simulink model "MLP_Final_Golden"  (R2015b)
settings: Solver=FixedStepDiscrete  SolverMode=SingleTasking  StartTime=0.0  StopTime=1e-2  RelTol=1e-3
undefined symbols (not defined in the file): input_sample_time, system_sample_time
libraries: shlslibv1 x1948
(part 1 of 11)
settings Model: synDspstartup=OK  Creator=txia13  LastModifiedBy=sshi23
settings DataIOCC: SaveOutput=off  SignalLogging=off  SaveTime=off
settings OptimizationCC: DefaultParameterBehavior=Inlined
settings DebuggingCC: AlgebraicLoopMsg=error  InheritedTsInSrcMsg=none

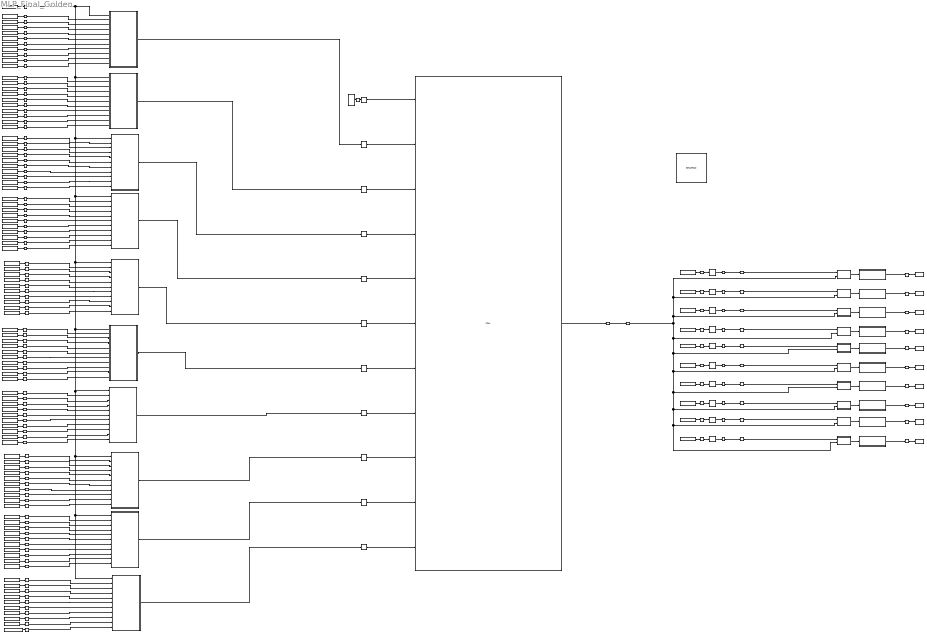
== system MLP_Final_Golden ==
  "Activation_Preparation_LoopLatency10 " : Subsystem
  Activation_Preparation_LoopLatency10 1 : Subsystem
  Activation_Preparation_LoopLatency10 2 : Subsystem
  Activation_Preparation_LoopLatency10 3 : Subsystem
  Activation_Preparation_LoopLatency10 4 : Subsystem
  Activation_Preparation_LoopLatency10 5 : Subsystem
  Activation_Preparation_LoopLatency10 6 : Subsystem
  Activation_Preparation_LoopLatency10 7 : Subsystem
  Activation_Preparation_LoopLatency10 8 : Subsystem
  Activation_Preparation_LoopLatency10 9 : Subsystem
  Counter : shlslibv1/Sources/Counter  syn_rst_port=off  syn_en_port=off  syn_ld_port=off  syn_cnt_type=Up  syn_init_val=0  syn_term_exists=on  syn_rdy_port=off  syn_term_val=9  syn_cnt_f=Automatic  syn_cnt_wl=8  syn_cnt_dt=unsigned  syn_cnt_st=BMUX_sample_time  synBlockType=primitive  synLatency=0  synBlockId=21
  Delay{1..10,21} (11 alike) : shlslibv1/Memories/Delay  syn_delay_val=7891  synBlockType=primitive  synLatency=7891  synBlockId=104
  Delay11 : shlslibv1/Memories/Delay  syn_delay_val=2  synBlockType=primitive  synLatency=2  synBlockId=104
  Delay12 : shlslibv1/Memories/Delay  syn_delay_val=12  synBlockType=primitive  synLatency=12  synBlockId=104
  Delay13 : shlslibv1/Memories/Delay  syn_delay_val=22  synBlockType=primitive  synLatency=22  synBlockId=104
  Delay14 : shlslibv1/Memories/Delay  syn_delay_val=32  synBlockType=primitive  synLatency=32  synBlockId=104
  Delay15 : shlslibv1/Memories/Delay  syn_delay_val=42  synBlockType=primitive  synLatency=42  synBlockId=104
  Delay16 : shlslibv1/Memories/Delay  syn_delay_val=52  synBlockType=primitive  synLatency=52  synBlockId=104
  Delay17 : shlslibv1/Memories/Delay  syn_delay_val=62  synBlockType=primitive  synLatency=62  synBlockId=104
  Delay18 : shlslibv1/Memories/Delay  syn_delay_val=72  synBlockType=primitive  synLatency=72  synBlockId=104
  Delay19 : shlslibv1/Memories/Delay  syn_delay_val=82  synBlockType=primitive  synLatency=82  synBlockId=104
  Delay20 : shlslibv1/Memories/Delay  syn_delay_val=92  synBlockType=primitive  synLatency=92  synBlockId=104
  From Workspace : FromWorkspace  VariableName=Input_Layer  SampleTime=input_sample_time  OutputAfterFinalValue=Setting to zero
  From Workspace1 : FromWorkspace  VariableName=Hidden_Layer_Weight1  SampleTime=input_sample_time  OutputAfterFinalValue=Setting to zero
  From Workspace10 : FromWorkspace  VariableName=Hidden_Layer_Weight5  SampleTime=input_sample_time  OutputAfterFinalValue=Setting to zero
  From Workspace102 : FromWorkspace  VariableName=Hidden_Layer_Weight51  SampleTime=input_sample_time  OutputAfterFinalValue=Setting to zero
  From Workspace103 : FromWorkspace  VariableName=Hidden_Layer_Weight55  SampleTime=input_sample_time  OutputAfterFinalValue=Setting to zero
  From Workspace106 : FromWorkspace  VariableName=Hidden_Layer_Weight56  SampleTime=input_sample_time  OutputAfterFinalValue=Setting to zero
  From Workspace107 : FromWorkspace  VariableName=Hidden_Layer_Weight58  SampleTime=input_sample_time  OutputAfterFinalValue=Setting to zero
  From Workspace109 : FromWorkspace  VariableName=Hidden_Layer_Weight59  SampleTime=input_sample_time  OutputAfterFinalValue=Setting to zero
  From Workspace111 : FromWorkspace  VariableName=Hidden_Layer_Weight57  SampleTime=input_sample_time  OutputAfterFinalValue=Setting to zero
  From Workspace114 : FromWorkspace  VariableName=Hidden_Layer_Weight60  SampleTime=input_sample_time  OutputAfterFinalValue=Setting to zero
  From Workspace116 : FromWorkspace  VariableName=Hidden_Layer_Weight61  SampleTime=input_sample_time  OutputAfterFinalValue=Setting to zero
  From Workspace117 : FromWorkspace  VariableName=Hidden_Layer_Weight65  SampleTime=input_sample_time  OutputAfterFinalValue=Setting to zero
  From Workspace119 : FromWorkspace  VariableName=Hidden_Layer_Weight66  SampleTime=input_sample_time  OutputAfterFinalValue=Setting to zero
  From Workspace12 : FromWorkspace  VariableName=Hidden_Layer_Weight6  SampleTime=input_sample_time  OutputAfterFinalValue=Setting to zero
  From Workspace120 : FromWorkspace  VariableName=Hidden_Layer_Weight68  SampleTime=input_sample_time  OutputAfterFinalValue=Setting to zero
  From Workspace122 : FromWorkspace  VariableName=Hidden_Layer_Weight69  SampleTime=input_sample_time  OutputAfterFinalValue=Setting to zero
  From Workspace125 : FromWorkspace  VariableName=Hidden_Layer_Weight67  SampleTime=input_sample_time  OutputAfterFinalValue=Setting to zero
  From Workspace128 : FromWorkspace  VariableName=Hidden_Layer_Weight70  SampleTime=input_sample_time  OutputAfterFinalValue=Setting to zero
  From Workspace13 : FromWorkspace  VariableName=Hidden_Layer_Weight8  SampleTime=input_sample_time  OutputAfterFinalValue=Setting to zero
  From Workspace130 : FromWorkspace  VariableName=Hidden_Layer_Weight62  SampleTime=input_sample_time  OutputAfterFinalValue=Setting to zero
  From Workspace132 : FromWorkspace  VariableName=Hidden_Layer_Weight63  SampleTime=input_sample_time  OutputAfterFinalValue=Setting to zero
  From Workspace134 : FromWorkspace  VariableName=Hidden_Layer_Weight64  SampleTime=input_sample_time  OutputAfterFinalValue=Setting to zero
  From Workspace135 : FromWorkspace  VariableName=Hidden_Layer_Weight52  SampleTime=input_sample_time  OutputAfterFinalValue=Setting to zero
  From Workspace138 : FromWorkspace  VariableName=Hidden_Layer_Weight71  SampleTime=input_sample_time  OutputAfterFinalValue=Setting to zero
  From Workspace139 : FromWorkspace  VariableName=Hidden_Layer_Weight75  SampleTime=input_sample_time  OutputAfterFinalValue=Setting to zero
  From Workspace141 : FromWorkspace  VariableName=Hidden_Layer_Weight76  SampleTime=input_sample_time  OutputAfterFinalValue=Setting to zero
  From Workspace142 : FromWorkspace  VariableName=Hidden_Layer_Weight78  SampleTime=input_sample_time  OutputAfterFinalValue=Setting to zero
  From Workspace144 : FromWorkspace  VariableName=Hidden_Layer_Weight79  SampleTime=input_sample_time  OutputAfterFinalValue=Setting to zero
  From Workspace147 : FromWorkspace  VariableName=Hidden_Layer_Weight77  SampleTime=input_sample_time  OutputAfterFinalValue=Setting to zero
  From Workspace15 : FromWorkspace  VariableName=Hidden_Layer_Weight9  SampleTime=input_sample_time  OutputAfterFinalValue=Setting to zero
  From Workspace150 : FromWorkspace  VariableName=Hidden_Layer_Weight80  SampleTime=input_sample_time  OutputAfterFinalValue=Setting to zero
  From Workspace152 : FromWorkspace  VariableName=Hidden_Layer_Weight72  SampleTime=input_sample_time  OutputAfterFinalValue=Setting to zero
  From Workspace154 : FromWorkspace  VariableName=Hidden_Layer_Weight73  SampleTime=input_sample_time  OutputAfterFinalValue=Setting to zero
  From Workspace156 : FromWorkspace  VariableName=Hidden_Layer_Weight74  SampleTime=input_sample_time  OutputAfterFinalValue=Setting to zero
  From Workspace157 : FromWorkspace  VariableName=Hidden_Layer_Weight53  SampleTime=input_sample_time  OutputAfterFinalValue=Setting to zero
  From Workspace160 : FromWorkspace  VariableName=Hidden_Layer_Weight81  SampleTime=input_sample_time  OutputAfterFinalValue=Setting to zero
  From Workspace161 : FromWorkspace  VariableName=Hidden_Layer_Weight85  SampleTime=input_sample_time  OutputAfterFinalValue=Setting to zero
  From Workspace163 : FromWorkspace  VariableName=Hidden_Layer_Weight86  SampleTime=input_sample_time  OutputAfterFinalValue=Setting to zero
  From Workspace164 : FromWorkspace  VariableName=Hidden_Layer_Weight88  SampleTime=input_sample_time  OutputAfterFinalValue=Setting to zero
  From Workspace166 : FromWorkspace  VariableName=Hidden_Layer_Weight89  SampleTime=input_sample_time  OutputAfterFinalValue=Setting to zero
  From Workspace169 : FromWorkspace  VariableName=Hidden_Layer_Weight87  SampleTime=input_sample_time  OutputAfterFinalValue=Setting to zero
  From Workspace17 : FromWorkspace  VariableName=Hidden_Layer_Weight7  SampleTime=input_sample_time  OutputAfterFinalValue=Setting to zero
  From Workspace172 : FromWorkspace  VariableName=Hidden_Layer_Weight90  SampleTime=input_sample_time  OutputAfterFinalValue=Setting to zero
  From Workspace174 : FromWorkspace  VariableName=Hidden_Layer_Weight82  SampleTime=input_sample_time  OutputAfterFinalValue=Setting to zero
  From Workspace176 : FromWorkspace  VariableName=Hidden_Layer_Weight83  SampleTime=input_sample_time  OutputAfterFinalValue=Setting to zero
  From Workspace178 : FromWorkspace  VariableName=Hidden_Layer_Weight84  SampleTime=input_sample_time  OutputAfterFinalValue=Setting to zero
  From Workspace179 : FromWorkspace  VariableName=Hidden_Layer_Weight54  SampleTime=input_sample_time  OutputAfterFinalValue=Setting to zero
  From Workspace182 : FromWorkspace  VariableName=Hidden_Layer_Weight91  SampleTime=input_sample_time  OutputAfterFinalValue=Setting to zero
  From Workspace183 : FromWorkspace  VariableName=Hidden_Layer_Weight95  SampleTime=input_sample_time  OutputAfterFinalValue=Setting to zero
  From Workspace185 : FromWorkspace  VariableName=Hidden_Layer_Weight96  SampleTime=input_sample_time  OutputAfterFinalValue=Setting to zero
  From Workspace186 : FromWorkspace  VariableName=Hidden_Layer_Weight98  SampleTime=input_sample_time  OutputAfterFinalValue=Setting to zero
  From Workspace188 : FromWorkspace  VariableName=Hidden_Layer_Weight99  SampleTime=input_sample_time  OutputAfterFinalValue=Setting to zero
  From Workspace191 : FromWorkspace  VariableName=Hidden_Layer_Weight97  SampleTime=input_sample_time  OutputAfterFinalValue=Setting to zero
  From Workspace194 : FromWorkspace  VariableName=Hidden_Layer_Weight100  SampleTime=input_sample_time  OutputAfterFinalValue=Setting to zero
  From Workspace196 : FromWorkspace  VariableName=Hidden_Layer_Weight92  SampleTime=input_sample_time  OutputAfterFinalValue=Setting to zero
  From Workspace198 : FromWorkspace  VariableName=Hidden_Layer_Weight93  SampleTime=input_sample_time  OutputAfterFinalValue=Setting to zero
  From Workspace2 : FromWorkspace  VariableName=Output_Layer_Weight1  SampleTime=system_sample_time  OutputAfterFinalValue=Setting to zero
  From Workspace20 : FromWorkspace  VariableName=Hidden_Layer_Weight10  SampleTime=input_sample_time  OutputAfterFinalValue=Setting to zero
  From Workspace200 : FromWorkspace  VariableName=Hidden_Layer_Weight94  SampleTime=input_sample_time  OutputAfterFinalValue=Setting to zero
  From Workspace201 : FromWorkspace  VariableName=Output_Layer_Weight2  SampleTime=system_sample_time  OutputAfterFinalValue=Setting to zero
  From Workspace202 : FromWorkspace  VariableName=Output_Layer_Weight3  SampleTime=input_sample_time  OutputAfterFinalValue=Setting to zero
  From Workspace203 : FromWorkspace  VariableName=Output_Layer_Weight4  SampleTime=system_sample_time  OutputAfterFinalValue=Setting to zero
  From Workspace204 : FromWorkspace  VariableName=Output_Layer_Weight5  SampleTime=system_sample_time  OutputAfterFinalValue=Setting to zero
  From Workspace205 : FromWorkspace  VariableName=Output_Layer_Weight6  SampleTime=system_sample_time  OutputAfterFinalValue=Setting to zero
  From Workspace206 : FromWorkspace  VariableName=Output_Layer_Weight7  SampleTime=system_sample_time  OutputAfterFinalValue=Setting to zero
  From Workspace207 : FromWorkspace  VariableName=Output_Layer_Weight8  SampleTime=system_sample_time  OutputAfterFinalValue=Setting to zero
  From Workspace208 : FromWorkspace  VariableName=Output_Layer_Weight9  SampleTime=system_sample_time  OutputAfterFinalValue=Setting to zero
  From Workspace209 : FromWorkspace  VariableName=Output_Layer_Weight10  SampleTime=input_sample_time  OutputAfterFinalValue=Setting to zero
  From Workspace22 : FromWorkspace  VariableName=Hidden_Layer_Weight11  SampleTime=input_sample_time  OutputAfterFinalValue=Setting to zero
  From Workspace23 : FromWorkspace  VariableName=Hidden_Layer_Weight15  SampleTime=input_sample_time  OutputAfterFinalValue=Setting to zero
  From Workspace25 : FromWorkspace  VariableName=Hidden_Layer_Weight16  SampleTime=input_sample_time  OutputAfterFinalValue=Setting to zero
  From Workspace26 : FromWorkspace  VariableName=Hidden_Layer_Weight18  SampleTime=input_sample_time  OutputAfterFinalValue=Setting to zero
  From Workspace28 : FromWorkspace  VariableName=Hidden_Layer_Weight19  SampleTime=input_sample_time  OutputAfterFinalValue=Setting to zero
  From Workspace30 : FromWorkspace  VariableName=Hidden_Layer_Weight17  SampleTime=input_sample_time  OutputAfterFinalValue=Setting to zero
  From Workspace33 : FromWorkspace  VariableName=Hidden_Layer_Weight20  SampleTime=input_sample_time  OutputAfterFinalValue=Setting to zero
  From Workspace35 : FromWorkspace  VariableName=Hidden_Layer_Weight12  SampleTime=input_sample_time  OutputAfterFinalValue=Setting to zero
  From Workspace37 : FromWorkspace  VariableName=Hidden_Layer_Weight13  SampleTime=input_sample_time  OutputAfterFinalValue=Setting to zero
  From Workspace39 : FromWorkspace  VariableName=Hidden_Layer_Weight14  SampleTime=input_sample_time  OutputAfterFinalValue=Setting to zero
  From Workspace4 : FromWorkspace  VariableName=Hidden_Layer_Weight2  SampleTime=input_sample_time  OutputAfterFinalValue=Setting to zero
  From Workspace42 : FromWorkspace  VariableName=Hidden_Layer_Weight21  SampleTime=input_sample_time  OutputAfterFinalValue=Setting to zero
  From Workspace43 : FromWorkspace  VariableName=Hidden_Layer_Weight25  SampleTime=input_sample_time  OutputAfterFinalValue=Setting to zero
  From Workspace45 : FromWorkspace  VariableName=Hidden_Layer_Weight26  SampleTime=input_sample_time  OutputAfterFinalValue=Setting to zero
  From Workspace46 : FromWorkspace  VariableName=Hidden_Layer_Weight28  SampleTime=input_sample_time  OutputAfterFinalValue=Setting to zero
  From Workspace48 : FromWorkspace  VariableName=Hidden_Layer_Weight29  SampleTime=input_sample_time  OutputAfterFinalValue=Setting to zero
  From Workspace50 : FromWorkspace  VariableName=Hidden_Layer_Weight27  SampleTime=input_sample_time  OutputAfterFinalValue=Setting to zero
  From Workspace53 : FromWorkspace  VariableName=Hidden_Layer_Weight30  SampleTime=input_sample_time  OutputAfterFinalValue=Setting to zero
  From Workspace55 : FromWorkspace  VariableName=Hidden_Layer_Weight22  SampleTime=input_sample_time  OutputAfterFinalValue=Setting to zero
  From Workspace57 : FromWorkspace  VariableName=Hidden_Layer_Weight23  SampleTime=input_sample_time  OutputAfterFinalValue=Setting to zero
  From Workspace59 : FromWorkspace  VariableName=Hidden_Layer_Weight24  SampleTime=input_sample_time  OutputAfterFinalValue=Setting to zero
  From Workspace6 : FromWorkspace  VariableName=Hidden_Layer_Weight3  SampleTime=input_sample_time  OutputAfterFinalValue=Setting to zero
  From Workspace62 : FromWorkspace  VariableName=Hidden_Layer_Weight31  SampleTime=input_sample_time  OutputAfterFinalValue=Setting to zero
  From Workspace63 : FromWorkspace  VariableName=Hidden_Layer_Weight35  SampleTime=input_sample_time  OutputAfterFinalValue=Setting to zero
  From Workspace65 : FromWorkspace  VariableName=Hidden_Layer_Weight36  SampleTime=input_sample_time  OutputAfterFinalValue=Setting to zero
  From Workspace66 : FromWorkspace  VariableName=Hidden_Layer_Weight38  SampleTime=input_sample_time  OutputAfterFinalValue=Setting to zero
  From Workspace68 : FromWorkspace  VariableName=Hidden_Layer_Weight39  SampleTime=input_sample_time  OutputAfterFinalValue=Setting to zero
  From Workspace70 : FromWorkspace  VariableName=Hidden_Layer_Weight37  SampleTime=input_sample_time  OutputAfterFinalValue=Setting to zero
  From Workspace73 : FromWorkspace  VariableName=Hidden_Layer_Weight40  SampleTime=input_sample_time  OutputAfterFinalValue=Setting to zero
  From Workspace75 : FromWorkspace  VariableName=Hidden_Layer_Weight32  SampleTime=input_sample_time  OutputAfterFinalValue=Setting to zero
  From Workspace77 : FromWorkspace  VariableName=Hidden_Layer_Weight33  SampleTime=input_sample_time  OutputAfterFinalValue=Setting to zero
  From Workspace79 : FromWorkspace  VariableName=Hidden_Layer_Weight34  SampleTime=input_sample_time  OutputAfterFinalValue=Setting to zero
  From Workspace8 : FromWorkspace  VariableName=Hidden_Layer_Weight4  SampleTime=input_sample_time  OutputAfterFinalValue=Setting to zero
  From Workspace82 : FromWorkspace  VariableName=Hidden_Layer_Weight41  SampleTime=input_sample_time  OutputAfterFinalValue=Setting to zero
  From Workspace83 : FromWorkspace  VariableName=Hidden_Layer_Weight45  SampleTime=input_sample_time  OutputAfterFinalValue=Setting to zero
  From Workspace85 : FromWorkspace  VariableName=Hidden_Layer_Weight46  SampleTime=input_sample_time  OutputAfterFinalValue=Setting to zero
  From Workspace86 : FromWorkspace  VariableName=Hidden_Layer_Weight48  SampleTime=input_sample_time  OutputAfterFinalValue=Setting to zero
  From Workspace88 : FromWorkspace  VariableName=Hidden_Layer_Weight49  SampleTime=input_sample_time  OutputAfterFinalValue=Setting to zero
  From Workspace90 : FromWorkspace  VariableName=Hidden_Layer_Weight47  SampleTime=input_sample_time  OutputAfterFinalValue=Setting to zero
  From Workspace93 : FromWorkspace  VariableName=Hidden_Layer_Weight50  SampleTime=input_sample_time  OutputAfterFinalValue=Setting to zero
  From Workspace95 : FromWorkspace  VariableName=Hidden_Layer_Weight42  SampleTime=input_sample_time  OutputAfterFinalValue=Setting to zero
  From Workspace97 : FromWorkspace  VariableName=Hidden_Layer_Weight43  SampleTime=input_sample_time  OutputAfterFinalValue=Setting to zero
  From Workspace99 : FromWorkspace  VariableName=Hidden_Layer_Weight44  SampleTime=input_sample_time  OutputAfterFinalValue=Setting to zero
  Mux : shlslibv1/Signal Operations/Mux  syn_in_nb=10  syn_out_f=Specify  syn_out_wl=32  syn_out_fl=16  syn_out_dt=unsigned  syn_en_se=off  synBlockType=primitive  synLatency=0  synBlockId=16
  New_Activation_Gold : Subsystem
  New_Activation_Gold1 : Subsystem
  New_Activation_Gold2 : Subsystem
  New_Activation_Gold3 : Subsystem
  New_Activation_Gold4 : Subsystem
  New_Activation_Gold5 : Subsystem
  New_Activation_Gold6 : Subsystem
  New_Activation_Gold7 : Subsystem
  New_Activation_Gold8 : Subsystem
  New_Activation_Gold9 : Subsystem
  Port In{,102..103,105,107,109,112,114,116,118,120} (11 alike) : shlslibv1/Ports & Subsystems/Port In  syn_out_wl=32  syn_out_fl=16  syn_out_dt=signed  syn_out_st=system_sample_time  syn_capture=on  syn_register=on  syn_out_sat=off  syn_out_rnd=on  synBlockType=port  synLatency=1  synBlockId=0
  Port In{1..100} (100 alike) : shlslibv1/Ports & Subsystems/Port In  syn_out_wl=32  syn_out_fl=16  syn_out_dt=signed  syn_out_st=input_sample_time  syn_capture=on  syn_register=on  syn_out_sat=off  syn_out_rnd=on  synBlockType=port  synLatency=1  synBlockId=0
  Port In{101,104,106,108,110..111,113,115,117,119,121} (11 alike) : shlslibv1/Ports & Subsystems/Port In  syn_out_wl=32  syn_out_fl=16  syn_out_dt=signed  syn_out_st=system_sample_time2  syn_capture=on  syn_register=on  syn_out_sat=off  syn_out_rnd=on  synBlockType=port  synLatency=1  synBlockId=0
  Port In210 : shlslibv1/Ports & Subsystems/Port In  syn_out_wl=32  syn_out_fl=16  syn_out_dt=unsigned  syn_out_st=system_sample_time  syn_capture=on  syn_register=on  syn_out_sat=off  syn_out_rnd=on  synBlockType=port  synLatency=1  synBlockId=0
  Port Out{,1..18,22..23} (21 alike) : shlslibv1/Ports & Subsystems/Port Out  syn_capture=on  syn_register=on  synBlockType=port  synLatency=1  synBlockId=1
  SHLSTool : shlslibv1/SHLSTool  synBlockType=tool  syn_dsp_mode=FPGA
  Subsystem : Subsystem
  Subsystem1 : Subsystem
  Subsystem2 : Subsystem
  Subsystem3 : Subsystem
  Subsystem4 : Subsystem
  Subsystem5 : Subsystem
  Subsystem6 : Subsystem
  Subsystem7 : Subsystem
  Subsystem8 : Subsystem
  Subsystem9 : Subsystem
  To Workspace : ToWorkspace  VariableName=Number0  SaveFormat=Structure With Time  SampleTime=-1
  To Workspace1 : ToWorkspace  VariableName=Number1  SaveFormat=Structure With Time  SampleTime=-1
  To Workspace2 : ToWorkspace  VariableName=Number2  SaveFormat=Structure With Time  SampleTime=-1
  To Workspace3 : ToWorkspace  VariableName=Number3  SaveFormat=Structure With Time  SampleTime=-1
  To Workspace4 : ToWorkspace  VariableName=Number4  SaveFormat=Structure With Time  SampleTime=-1
  To Workspace5 : ToWorkspace  VariableName=Number5  SaveFormat=Structure With Time  SampleTime=-1
  To Workspace6 : ToWorkspace  VariableName=Number6  SaveFormat=Structure With Time  SampleTime=-1
  To Workspace7 : ToWorkspace  VariableName=Number7  SaveFormat=Structure With Time  SampleTime=-1
  To Workspace8 : ToWorkspace  VariableName=Number8  SaveFormat=Structure With Time  SampleTime=-1
  To Workspace9 : ToWorkspace  VariableName=Number9  SaveFormat=Structure With Time  SampleTime=-1
  wires:
  From Workspace/1 -> Port In/1
  From Workspace1/1 -> Port In1/1
  From Workspace4/1 -> Port In2/1
  From Workspace6/1 -> Port In3/1
  From Workspace8/1 -> Port In4/1
  From Workspace10/1 -> Port In5/1
  From Workspace12/1 -> Port In6/1
  From Workspace17/1 -> Port In7/1
  From Workspace13/1 -> Port In8/1
  From Workspace15/1 -> Port In9/1
  From Workspace20/1 -> Port In10/1
  Subsystem/1(Out1) -> Delay11/1
  From Workspace22/1 -> Port In11/1
  From Workspace35/1 -> Port In12/1
  From Workspace37/1 -> Port In13/1
  From Workspace39/1 -> Port In14/1
  From Workspace23/1 -> Port In15/1
  From Workspace25/1 -> Port In16/1
  From Workspace30/1 -> Port In17/1
  From Workspace26/1 -> Port In18/1
  From Workspace28/1 -> Port In19/1
  From Workspace33/1 -> Port In20/1
  Subsystem1/1(Out1) -> Delay12/1
  From Workspace42/1 -> Port In21/1
  From Workspace55/1 -> Port In22/1
  From Workspace57/1 -> Port In23/1
  From Workspace59/1 -> Port In24/1
  From Workspace43/1 -> Port In25/1
  From Workspace45/1 -> Port In26/1
  From Workspace50/1 -> Port In27/1
  From Workspace46/1 -> Port In28/1
  From Workspace48/1 -> Port In29/1
  From Workspace53/1 -> Port In30/1
  From Workspace62/1 -> Port In31/1
  From Workspace75/1 -> Port In32/1
  From Workspace77/1 -> Port In33/1
  From Workspace79/1 -> Port In34/1
  From Workspace63/1 -> Port In35/1
  From Workspace65/1 -> Port In36/1
  From Workspace70/1 -> Port In37/1
  From Workspace66/1 -> Port In38/1
  From Workspace68/1 -> Port In39/1
  From Workspace73/1 -> Port In40/1
  From Workspace82/1 -> Port In41/1
  From Workspace95/1 -> Port In42/1
  From Workspace97/1 -> Port In43/1
  From Workspace99/1 -> Port In44/1
  From Workspace83/1 -> Port In45/1
  From Workspace85/1 -> Port In46/1
  From Workspace90/1 -> Port In47/1
  From Workspace86/1 -> Port In48/1
  From Workspace88/1 -> Port In49/1
  From Workspace93/1 -> Port In50/1
  From Workspace102/1 -> Port In51/1
  From Workspace135/1 -> Port In52/1
  From Workspace157/1 -> Port In53/1
  From Workspace179/1 -> Port In54/1
  From Workspace103/1 -> Port In55/1
  From Workspace106/1 -> Port In56/1
  From Workspace111/1 -> Port In57/1
  From Workspace107/1 -> Port In58/1
  From Workspace109/1 -> Port In59/1
  From Workspace114/1 -> Port In60/1
  From Workspace116/1 -> Port In61/1
  From Workspace130/1 -> Port In62/1
  From Workspace132/1 -> Port In63/1
  From Workspace134/1 -> Port In64/1
  From Workspace117/1 -> Port In65/1
  From Workspace119/1 -> Port In66/1
  From Workspace125/1 -> Port In67/1
  From Workspace120/1 -> Port In68/1
  From Workspace122/1 -> Port In69/1
  From Workspace128/1 -> Port In70/1
  From Workspace138/1 -> Port In71/1
  From Workspace152/1 -> Port In72/1
  From Workspace154/1 -> Port In73/1
  From Workspace156/1 -> Port In74/1
  From Workspace139/1 -> Port In75/1
  From Workspace141/1 -> Port In76/1
  From Workspace147/1 -> Port In77/1
  From Workspace142/1 -> Port In78/1
  From Workspace144/1 -> Port In79/1
  From Workspace150/1 -> Port In80/1
  From Workspace160/1 -> Port In81/1
  From Workspace174/1 -> Port In82/1
  From Workspace176/1 -> Port In83/1
  From Workspace178/1 -> Port In84/1
  From Workspace161/1 -> Port In85/1
  From Workspace163/1 -> Port In86/1
  From Workspace169/1 -> Port In87/1
  From Workspace164/1 -> Port In88/1
  From Workspace166/1 -> Port In89/1
  From Workspace172/1 -> Port In90/1
  From Workspace182/1 -> Port In91/1
  From Workspace196/1 -> Port In92/1
  From Workspace198/1 -> Port In93/1
  From Workspace200/1 -> Port In94/1
  From Workspace183/1 -> Port In95/1
  From Workspace185/1 -> Port In96/1
  From Workspace191/1 -> Port In97/1
  From Workspace186/1 -> Port In98/1
  From Workspace188/1 -> Port In99/1
  From Workspace194/1 -> Port In100/1
  Subsystem2/1(Out1) -> Delay13/1
  Subsystem3/1(Out1) -> Delay14/1
  Subsystem4/1(Out1) -> Delay15/1
  Subsystem5/1(Out1) -> Delay16/1
  Subsystem6/1(Out1) -> Delay17/1
  Subsystem7/1(Out1) -> Delay18/1
  Subsystem8/1(Out1) -> Delay19/1
  Subsystem9/1(Out1) -> Delay20/1
  Delay21/1 -> Mux/1
  Counter/1 -> Port In210/1
  Port In210/1 -> Delay21/1
  Delay11/1 -> Mux/2
  Delay12/1 -> Mux/3
  Delay13/1 -> Mux/4
  Delay14/1 -> Mux/5
  Delay15/1 -> Mux/6
  Delay16/1 -> Mux/7
  Delay17/1 -> Mux/8
  Delay18/1 -> Mux/9
  Delay19/1 -> Mux/10
  Delay20/1 -> Mux/11
  Mux/1 -> Port Out22/1
  Port In1/1 -> Subsystem/2(In2)
  Port In2/1 -> Subsystem/3(In3)
  Port In3/1 -> Subsystem/4(In4)
  Port In4/1 -> Subsystem/5(In5)
  Port In5/1 -> Subsystem/6(In6)
  Port In6/1 -> Subsystem/7(In7)
  Port In7/1 -> Subsystem/8(In8)
  Port In8/1 -> Subsystem/9(In9)
  Port In9/1 -> Subsystem/10(In10)
  Port In10/1 -> Subsystem/11(In11)
  Port In/1 -> Subsystem1/1(In1), Subsystem2/1(In1), Subsystem3/1(In1), Subsystem4/1(In1), Subsystem5/1(In1), Subsystem6/1(In1), Subsystem7/1(In1), Subsystem9/1(In1), Subsystem8/1(In1), Subsystem/1(In1)
  Port In11/1 -> Subsystem1/2(In2)
  Port In12/1 -> Subsystem1/3(In3)
  Port In13/1 -> Subsystem1/4(In4)
  Port In14/1 -> Subsystem1/5(In5)
  Port In15/1 -> Subsystem1/6(In6)
  Port In16/1 -> Subsystem1/7(In7)
  Port In17/1 -> Subsystem1/8(In8)
  Port In18/1 -> Subsystem1/9(In9)
  Port In19/1 -> Subsystem1/10(In10)
  Port In20/1 -> Subsystem1/11(In11)
  Port In21/1 -> Subsystem2/2(In2)
  Port In22/1 -> Subsystem2/3(In3)
  Port In23/1 -> Subsystem2/4(In4)
  Port In24/1 -> Subsystem2/5(In5)
  Port In25/1 -> Subsystem2/6(In6)
  Port In26/1 -> Subsystem2/7(In7)
  Port In27/1 -> Subsystem2/8(In8)
  Port In28/1 -> Subsystem2/9(In9)
  Port In29/1 -> Subsystem2/10(In10)
  Port In30/1 -> Subsystem2/11(In11)
  Port In31/1 -> Subsystem3/2(In2)
  Port In32/1 -> Subsystem3/3(In3)
  Port In33/1 -> Subsystem3/4(In4)
  Port In34/1 -> Subsystem3/5(In5)
  Port In35/1 -> Subsystem3/6(In6)
  Port In36/1 -> Subsystem3/7(In7)
  Port In37/1 -> Subsystem3/8(In8)
  Port In38/1 -> Subsystem3/9(In9)
  Port In39/1 -> Subsystem3/10(In10)
  Port In40/1 -> Subsystem3/11(In11)
  Port In41/1 -> Subsystem4/2(In2)
  Port In42/1 -> Subsystem4/3(In3)
  Port In43/1 -> Subsystem4/4(In4)
  Port In44/1 -> Subsystem4/5(In5)
  Port In45/1 -> Subsystem4/6(In6)
  Port In46/1 -> Subsystem4/7(In7)
  Port In47/1 -> Subsystem4/8(In8)
  Port In48/1 -> Subsystem4/9(In9)
  Port In49/1 -> Subsystem4/10(In10)
  Port In50/1 -> Subsystem4/11(In11)
  Port In51/1 -> Subsystem5/2(In2)
  Port In52/1 -> Subsystem5/3(In3)
  Port In53/1 -> Subsystem5/4(In4)
  Port In54/1 -> Subsystem5/5(In5)
  Port In55/1 -> Subsystem5/6(In6)
  Port In56/1 -> Subsystem5/7(In7)
  Port In57/1 -> Subsystem5/8(In8)
  Port In58/1 -> Subsystem5/9(In9)
  Port In59/1 -> Subsystem5/10(In10)
  Port In60/1 -> Subsystem5/11(In11)
  Port In61/1 -> Subsystem6/2(In2)
  Port In62/1 -> Subsystem6/3(In3)
  Port In63/1 -> Subsystem6/4(In4)
  Port In64/1 -> Subsystem6/5(In5)
  Port In65/1 -> Subsystem6/6(In6)
  Port In66/1 -> Subsystem6/7(In7)
  Port In67/1 -> Subsystem6/8(In8)
  Port In68/1 -> Subsystem6/9(In9)
  Port In69/1 -> Subsystem6/10(In10)
  Port In70/1 -> Subsystem6/11(In11)
  Port In71/1 -> Subsystem7/2(In2)
  Port In72/1 -> Subsystem7/3(In3)
  Port In73/1 -> Subsystem7/4(In4)
  Port In74/1 -> Subsystem7/5(In5)
  Port In75/1 -> Subsystem7/6(In6)
  Port In76/1 -> Subsystem7/7(In7)
  Port In77/1 -> Subsystem7/8(In8)
  Port In78/1 -> Subsystem7/9(In9)
  Port In79/1 -> Subsystem7/10(In10)
  Port In80/1 -> Subsystem7/11(In11)
  Port In81/1 -> Subsystem8/2(In2)
  Port In82/1 -> Subsystem8/3(In3)
  Port In83/1 -> Subsystem8/4(In4)
  Port In84/1 -> Subsystem8/5(In5)
  Port In85/1 -> Subsystem8/6(In6)
  Port In86/1 -> Subsystem8/7(In7)
  Port In87/1 -> Subsystem8/8(In8)
  Port In88/1 -> Subsystem8/9(In9)
  Port In89/1 -> Subsystem8/10(In10)
  Port In90/1 -> Subsystem8/11(In11)
  Port In91/1 -> Subsystem9/2(In2)
  Port In92/1 -> Subsystem9/3(In3)
  Port In93/1 -> Subsystem9/4(In4)
  Port In94/1 -> Subsystem9/5(In5)
  Port In95/1 -> Subsystem9/6(In6)
  Port In96/1 -> Subsystem9/7(In7)
  Port In97/1 -> Subsystem9/8(In8)
  Port In98/1 -> Subsystem9/9(In9)
  Port In99/1 -> Subsystem9/10(In10)
  Port In100/1 -> Subsystem9/11(In11)
  Port In104/1 -> Activation_Preparation_LoopLatency10 5/1(In1)
  Port In110/1 -> Activation_Preparation_LoopLatency10 8/1(In1)
  Port In113/1 -> Activation_Preparation_LoopLatency10 9/1(In1)
  New_Activation_Gold/1(Out1) -> Port Out/1
  Port Out/1 -> To Workspace/1
  Port Out1/1 -> To Workspace1/1
  Port Out2/1 -> To Workspace2/1
  Port Out3/1 -> To Workspace3/1
  Port Out4/1 -> To Workspace4/1
  Port Out5/1 -> To Workspace5/1
  Port Out6/1 -> To Workspace6/1
  Port Out7/1 -> To Workspace7/1
  Port Out8/1 -> To Workspace8/1
  Port Out9/1 -> To Workspace9/1
  Delay1/1 -> Port Out23/1
  Port Out23/1 -> Port In111/1
  Port In103/1 -> Delay1/1
  From Workspace2/1 -> Port In103/1
  From Workspace201/1 -> Port In114/1
  From Workspace202/1 -> Port In116/1
  From Workspace203/1 -> Port In118/1
  From Workspace204/1 -> Port In120/1
  From Workspace205/1 -> Port In102/1
  From Workspace206/1 -> Port In105/1
  From Workspace208/1 -> Port In109/1
  From Workspace209/1 -> Port In112/1
  New_Activation_Gold9/1(Out1) -> Port Out9/1
  New_Activation_Gold8/1(Out1) -> Port Out8/1
  New_Activation_Gold7/1(Out1) -> Port Out7/1
  New_Activation_Gold1/1(Out1) -> Port Out1/1
  New_Activation_Gold2/1(Out1) -> Port Out2/1
  New_Activation_Gold3/1(Out1) -> Port Out3/1
  New_Activation_Gold4/1(Out1) -> Port Out4/1
  New_Activation_Gold5/1(Out1) -> Port Out5/1
  New_Activation_Gold6/1(Out1) -> Port Out6/1
  Port In115/1 -> Activation_Preparation_LoopLatency10 1/1(In1)
  Port In117/1 -> Activation_Preparation_LoopLatency10 2/1(In1)
  Port In119/1 -> Activation_Preparation_LoopLatency10 3/1(In1)
  Port In121/1 -> Activation_Preparation_LoopLatency10 4/1(In1)
  Port In106/1 -> Activation_Preparation_LoopLatency10 6/1(In1)
  From Workspace207/1 -> Port In107/1
  Port In108/1 -> Activation_Preparation_LoopLatency10 7/1(In1)
  Delay2/1 -> Port Out10/1
  Port Out10/1 -> Port In115/1
  Port In114/1 -> Delay2/1
  Delay3/1 -> Port Out11/1
  Port Out11/1 -> Port In117/1
  Port In116/1 -> Delay3/1
  Delay4/1 -> Port Out12/1
  Port Out12/1 -> Port In119/1
  Port In118/1 -> Delay4/1
  Delay5/1 -> Port Out13/1
  Port Out13/1 -> Port In121/1
  Port In120/1 -> Delay5/1
  Delay6/1 -> Port Out14/1
  Port Out14/1 -> Port In104/1
  Port In102/1 -> Delay6/1
  Delay7/1 -> Port Out15/1
  Port Out15/1 -> Port In106/1
  Port In105/1 -> Delay7/1
  Delay8/1 -> Port Out16/1
  Port Out16/1 -> Port In108/1
  Port In107/1 -> Delay8/1
  Delay9/1 -> Port Out17/1
  Port Out17/1 -> Port In110/1
  Port In109/1 -> Delay9/1
  Delay10/1 -> Port Out18/1
  Port Out18/1 -> Port In113/1
  Port In112/1 -> Delay10/1
  "Activation_Preparation_LoopLatency10 "/1(Out1) -> New_Activation_Gold/1(In1)
  Activation_Preparation_LoopLatency10 1/1(Out1) -> New_Activation_Gold1/1(In1)
  Activation_Preparation_LoopLatency10 2/1(Out1) -> New_Activation_Gold2/1(In1)
  Activation_Preparation_LoopLatency10 3/1(Out1) -> New_Activation_Gold3/1(In1)
  Activation_Preparation_LoopLatency10 4/1(Out1) -> New_Activation_Gold4/1(In1)
  Activation_Preparation_LoopLatency10 5/1(Out1) -> New_Activation_Gold5/1(In1)
  Activation_Preparation_LoopLatency10 6/1(Out1) -> New_Activation_Gold6/1(In1)
  Activation_Preparation_LoopLatency10 7/1(Out1) -> New_Activation_Gold7/1(In1)
  Activation_Preparation_LoopLatency10 8/1(Out1) -> New_Activation_Gold8/1(In1)
  Activation_Preparation_LoopLatency10 9/1(Out1) -> New_Activation_Gold9/1(In1)
  Port In101/1 -> Activation_Preparation_LoopLatency10 4/2(In2), Activation_Preparation_LoopLatency10 5/2(In2), Activation_Preparation_LoopLatency10 6/2(In2), Activation_Preparation_LoopLatency10 7/2(In2), Activation_Preparation_LoopLatency10 9/2(In2), Activation_Preparation_LoopLatency10 8/2(In2), Activation_Preparation_LoopLatency10 3/2(In2), Activation_Preparation_LoopLatency10 2/2(In2), Activation_Preparation_LoopLatency10 1/2(In2), "Activation_Preparation_LoopLatency10 "/2(In2)
  Port In111/1 -> "Activation_Preparation_LoopLatency10 "/1(In1)
  Port Out22/1 -> Port In101/1

== system MLP_Final_Golden/Activation_Preparation_LoopLatency10  ==
  In1 : Inport
  In2 : Inport  Port=2
  Add : shlslibv1/Math Functions/Add  syn_add_opr=++  syn_out_f=Specify  syn_out_wl=32  syn_out_fl=16  syn_out_dt=signed  syn_out_sat=off  syn_out_rnd=Floor (Truncate)  synBlockType=primitive  synLatency=0  synBlockId=96  syn_sum_of_rows=off  syn_inh_port=off  syn_inh_st=on  syn_inh_stf=1  syn_en_pipe=on  syn_pipe_stg=9  syn_flow_ctrl=off
  Delay : shlslibv1/Memories/Delay  syn_delay_val=1  synBlockType=primitive  synLatency=1  synBlockId=104
  Mult : shlslibv1/Math Functions/Mult  syn_out_f=Specify  syn_out_wl=32  syn_out_fl=16  syn_out_dt=signed  syn_out_sat=off  syn_out_rnd=Floor (Truncate)  syn_inh_port=off  syn_inh_st=off  syn_inh_stf=1  syn_en_pipe=on  syn_pipe_stg=10  syn_flow_ctrl=off  synBlockType=primitive  synLatency=0  synBlockId=3  syn_opr_mode=1
  Out1 : Outport
  wires:
  Mult/1 -> Add/2
  In2/1 -> Mult/2
  Add/1 -> Out1/1, Delay/1
  Delay/1 -> Add/1
  In1/1 -> Mult/1

== system MLP_Final_Golden/Activation_Preparation_LoopLatency10 1 ==
  In1 : Inport
  In2 : Inport  Port=2
  Add : shlslibv1/Math Functions/Add  syn_add_opr=++  syn_out_f=Specify  syn_out_wl=32  syn_out_fl=16  syn_out_dt=signed  syn_out_sat=off  syn_out_rnd=Floor (Truncate)  synBlockType=primitive  synLatency=0  synBlockId=96  syn_sum_of_rows=off  syn_inh_port=off  syn_inh_st=on  syn_inh_stf=1  syn_en_pipe=on  syn_pipe_stg=9  syn_flow_ctrl=off
  Delay : shlslibv1/Memories/Delay  syn_delay_val=1  synBlockType=primitive  synLatency=1  synBlockId=104
  Mult : shlslibv1/Math Functions/Mult  syn_out_f=Specify  syn_out_wl=32  syn_out_fl=16  syn_out_dt=signed  syn_out_sat=off  syn_out_rnd=Floor (Truncate)  syn_inh_port=off  syn_inh_st=off  syn_inh_stf=1  syn_en_pipe=on  syn_pipe_stg=10  syn_flow_ctrl=off  synBlockType=primitive  synLatency=0  synBlockId=3  syn_opr_mode=1
  Out1 : Outport
  wires:
  Mult/1 -> Add/2
  In2/1 -> Mult/2
  Add/1 -> Out1/1, Delay/1
  Delay/1 -> Add/1
  In1/1 -> Mult/1

== system MLP_Final_Golden/Activation_Preparation_LoopLatency10 2 ==
  In1 : Inport
  In2 : Inport  Port=2
  Add : shlslibv1/Math Functions/Add  syn_add_opr=++  syn_out_f=Specify  syn_out_wl=32  syn_out_fl=16  syn_out_dt=signed  syn_out_sat=off  syn_out_rnd=Floor (Truncate)  synBlockType=primitive  synLatency=0  synBlockId=96  syn_sum_of_rows=off  syn_inh_port=off  syn_inh_st=on  syn_inh_stf=1  syn_en_pipe=on  syn_pipe_stg=9  syn_flow_ctrl=off
  Delay : shlslibv1/Memories/Delay  syn_delay_val=1  synBlockType=primitive  synLatency=1  synBlockId=104
  Mult : shlslibv1/Math Functions/Mult  syn_out_f=Specify  syn_out_wl=32  syn_out_fl=16  syn_out_dt=signed  syn_out_sat=off  syn_out_rnd=Floor (Truncate)  syn_inh_port=off  syn_inh_st=off  syn_inh_stf=1  syn_en_pipe=on  syn_pipe_stg=10  syn_flow_ctrl=off  synBlockType=primitive  synLatency=0  synBlockId=3  syn_opr_mode=1
  Out1 : Outport
  wires:
  Mult/1 -> Add/2
  In2/1 -> Mult/2
  Add/1 -> Out1/1, Delay/1
  Delay/1 -> Add/1
  In1/1 -> Mult/1

== system MLP_Final_Golden/Activation_Preparation_LoopLatency10 3 ==
  In1 : Inport
  In2 : Inport  Port=2
  Add : shlslibv1/Math Functions/Add  syn_add_opr=++  syn_out_f=Specify  syn_out_wl=32  syn_out_fl=16  syn_out_dt=signed  syn_out_sat=off  syn_out_rnd=Floor (Truncate)  synBlockType=primitive  synLatency=0  synBlockId=96  syn_sum_of_rows=off  syn_inh_port=off  syn_inh_st=on  syn_inh_stf=1  syn_en_pipe=on  syn_pipe_stg=9  syn_flow_ctrl=off
  Delay : shlslibv1/Memories/Delay  syn_delay_val=1  synBlockType=primitive  synLatency=1  synBlockId=104
  Mult : shlslibv1/Math Functions/Mult  syn_out_f=Specify  syn_out_wl=32  syn_out_fl=16  syn_out_dt=signed  syn_out_sat=off  syn_out_rnd=Floor (Truncate)  syn_inh_port=off  syn_inh_st=off  syn_inh_stf=1  syn_en_pipe=on  syn_pipe_stg=10  syn_flow_ctrl=off  synBlockType=primitive  synLatency=0  synBlockId=3  syn_opr_mode=1
  Out1 : Outport
  wires:
  Mult/1 -> Add/2
  In2/1 -> Mult/2
  Add/1 -> Out1/1, Delay/1
  Delay/1 -> Add/1
  In1/1 -> Mult/1

== system MLP_Final_Golden/Activation_Preparation_LoopLatency10 4 ==
  In1 : Inport
  In2 : Inport  Port=2
  Add : shlslibv1/Math Functions/Add  syn_add_opr=++  syn_out_f=Specify  syn_out_wl=32  syn_out_fl=16  syn_out_dt=signed  syn_out_sat=off  syn_out_rnd=Floor (Truncate)  synBlockType=primitive  synLatency=0  synBlockId=96  syn_sum_of_rows=off  syn_inh_port=off  syn_inh_st=on  syn_inh_stf=1  syn_en_pipe=on  syn_pipe_stg=9  syn_flow_ctrl=off
  Delay : shlslibv1/Memories/Delay  syn_delay_val=1  synBlockType=primitive  synLatency=1  synBlockId=104
  Mult : shlslibv1/Math Functions/Mult  syn_out_f=Specify  syn_out_wl=32  syn_out_fl=16  syn_out_dt=signed  syn_out_sat=off  syn_out_rnd=Floor (Truncate)  syn_inh_port=off  syn_inh_st=off  syn_inh_stf=1  syn_en_pipe=on  syn_pipe_stg=10  syn_flow_ctrl=off  synBlockType=primitive  synLatency=0  synBlockId=3  syn_opr_mode=1
  Out1 : Outport
  wires:
  Mult/1 -> Add/2
  In2/1 -> Mult/2
  Add/1 -> Out1/1, Delay/1
  Delay/1 -> Add/1
  In1/1 -> Mult/1

== system MLP_Final_Golden/Activation_Preparation_LoopLatency10 5 ==
  In1 : Inport
  In2 : Inport  Port=2
  Add : shlslibv1/Math Functions/Add  syn_add_opr=++  syn_out_f=Specify  syn_out_wl=32  syn_out_fl=16  syn_out_dt=signed  syn_out_sat=off  syn_out_rnd=Floor (Truncate)  synBlockType=primitive  synLatency=0  synBlockId=96  syn_sum_of_rows=off  syn_inh_port=off  syn_inh_st=on  syn_inh_stf=1  syn_en_pipe=on  syn_pipe_stg=9  syn_flow_ctrl=off
  Delay : shlslibv1/Memories/Delay  syn_delay_val=1  synBlockType=primitive  synLatency=1  synBlockId=104
  Mult : shlslibv1/Math Functions/Mult  syn_out_f=Specify  syn_out_wl=32  syn_out_fl=16  syn_out_dt=signed  syn_out_sat=off  syn_out_rnd=Floor (Truncate)  syn_inh_port=off  syn_inh_st=off  syn_inh_stf=1  syn_en_pipe=on  syn_pipe_stg=10  syn_flow_ctrl=off  synBlockType=primitive  synLatency=0  synBlockId=3  syn_opr_mode=1
  Out1 : Outport
  wires:
  Mult/1 -> Add/2
  In2/1 -> Mult/2
  Add/1 -> Out1/1, Delay/1
  Delay/1 -> Add/1
  In1/1 -> Mult/1

== system MLP_Final_Golden/Activation_Preparation_LoopLatency10 6 ==
  In1 : Inport
  In2 : Inport  Port=2
  Add : shlslibv1/Math Functions/Add  syn_add_opr=++  syn_out_f=Specify  syn_out_wl=32  syn_out_fl=16  syn_out_dt=signed  syn_out_sat=off  syn_out_rnd=Floor (Truncate)  synBlockType=primitive  synLatency=0  synBlockId=96  syn_sum_of_rows=off  syn_inh_port=off  syn_inh_st=on  syn_inh_stf=1  syn_en_pipe=on  syn_pipe_stg=9  syn_flow_ctrl=off
  Delay : shlslibv1/Memories/Delay  syn_delay_val=1  synBlockType=primitive  synLatency=1  synBlockId=104
  Mult : shlslibv1/Math Functions/Mult  syn_out_f=Specify  syn_out_wl=32  syn_out_fl=16  syn_out_dt=signed  syn_out_sat=off  syn_out_rnd=Floor (Truncate)  syn_inh_port=off  syn_inh_st=off  syn_inh_stf=1  syn_en_pipe=on  syn_pipe_stg=10  syn_flow_ctrl=off  synBlockType=primitive  synLatency=0  synBlockId=3  syn_opr_mode=1
  Out1 : Outport
  wires:
  Mult/1 -> Add/2
  In2/1 -> Mult/2
  Add/1 -> Out1/1, Delay/1
  Delay/1 -> Add/1
  In1/1 -> Mult/1

== system MLP_Final_Golden/Activation_Preparation_LoopLatency10 7 ==
  In1 : Inport
  In2 : Inport  Port=2
  Add : shlslibv1/Math Functions/Add  syn_add_opr=++  syn_out_f=Specify  syn_out_wl=32  syn_out_fl=16  syn_out_dt=signed  syn_out_sat=off  syn_out_rnd=Floor (Truncate)  synBlockType=primitive  synLatency=0  synBlockId=96  syn_sum_of_rows=off  syn_inh_port=off  syn_inh_st=on  syn_inh_stf=1  syn_en_pipe=on  syn_pipe_stg=9  syn_flow_ctrl=off
  Delay : shlslibv1/Memories/Delay  syn_delay_val=1  synBlockType=primitive  synLatency=1  synBlockId=104
  Mult : shlslibv1/Math Functions/Mult  syn_out_f=Specify  syn_out_wl=32  syn_out_fl=16  syn_out_dt=signed  syn_out_sat=off  syn_out_rnd=Floor (Truncate)  syn_inh_port=off  syn_inh_st=off  syn_inh_stf=1  syn_en_pipe=on  syn_pipe_stg=10  syn_flow_ctrl=off  synBlockType=primitive  synLatency=0  synBlockId=3  syn_opr_mode=1
  Out1 : Outport
  wires:
  Mult/1 -> Add/2
  In2/1 -> Mult/2
  Add/1 -> Out1/1, Delay/1
  Delay/1 -> Add/1
  In1/1 -> Mult/1

== system MLP_Final_Golden/Activation_Preparation_LoopLatency10 8 ==
  In1 : Inport
  In2 : Inport  Port=2
  Add : shlslibv1/Math Functions/Add  syn_add_opr=++  syn_out_f=Specify  syn_out_wl=32  syn_out_fl=16  syn_out_dt=signed  syn_out_sat=off  syn_out_rnd=Floor (Truncate)  synBlockType=primitive  synLatency=0  synBlockId=96  syn_sum_of_rows=off  syn_inh_port=off  syn_inh_st=on  syn_inh_stf=1  syn_en_pipe=on  syn_pipe_stg=9  syn_flow_ctrl=off
  Delay : shlslibv1/Memories/Delay  syn_delay_val=1  synBlockType=primitive  synLatency=1  synBlockId=104
  Mult : shlslibv1/Math Functions/Mult  syn_out_f=Specify  syn_out_wl=32  syn_out_fl=16  syn_out_dt=signed  syn_out_sat=off  syn_out_rnd=Floor (Truncate)  syn_inh_port=off  syn_inh_st=off  syn_inh_stf=1  syn_en_pipe=on  syn_pipe_stg=10  syn_flow_ctrl=off  synBlockType=primitive  synLatency=0  synBlockId=3  syn_opr_mode=1
  Out1 : Outport
  wires:
  Mult/1 -> Add/2
  In2/1 -> Mult/2
  Add/1 -> Out1/1, Delay/1
  Delay/1 -> Add/1
  In1/1 -> Mult/1

== system MLP_Final_Golden/Activation_Preparation_LoopLatency10 9 ==
  In1 : Inport
  In2 : Inport  Port=2
  Add : shlslibv1/Math Functions/Add  syn_add_opr=++  syn_out_f=Specify  syn_out_wl=32  syn_out_fl=16  syn_out_dt=signed  syn_out_sat=off  syn_out_rnd=Floor (Truncate)  synBlockType=primitive  synLatency=0  synBlockId=96  syn_sum_of_rows=off  syn_inh_port=off  syn_inh_st=on  syn_inh_stf=1  syn_en_pipe=on  syn_pipe_stg=9  syn_flow_ctrl=off
  Delay : shlslibv1/Memories/Delay  syn_delay_val=1  synBlockType=primitive  synLatency=1  synBlockId=104
  Mult : shlslibv1/Math Functions/Mult  syn_out_f=Specify  syn_out_wl=32  syn_out_fl=16  syn_out_dt=signed  syn_out_sat=off  syn_out_rnd=Floor (Truncate)  syn_inh_port=off  syn_inh_st=off  syn_inh_stf=1  syn_en_pipe=on  syn_pipe_stg=10  syn_flow_ctrl=off  synBlockType=primitive  synLatency=0  synBlockId=3  syn_opr_mode=1
  Out1 : Outport
  wires:
  Mult/1 -> Add/2
  In2/1 -> Mult/2
  Add/1 -> Out1/1, Delay/1
  Delay/1 -> Add/1
  In1/1 -> Mult/1
